simulink model "time_domain_exe2_not_autonomous"  (R2020b)
settings: Solver=VariableStepAuto  StartTime=0.0  StopTime=10.0  RelTol=1e-3
settings Model: Creator=petir  LastModifiedBy=petir

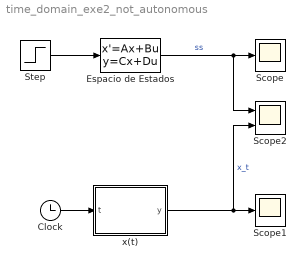
== system time_domain_exe2_not_autonomous ==
  Clock : Clock
  Espacio de Estados : StateSpace  A=[-5 0; 0 -5]  B=[5; 5]  C=[1, -1]  D=[0]  InitialCondition=[2; -1]
  Scope : Scope
  Scope1 : Scope
  Scope2 : Scope  NumInputPorts=2
  Step : Step  SampleTime=0
  x(t) : MATLAB Function  TreatAsAtomicUnit=on
  wires:
  Espacio de Estados/1 -> Scope2/1, Scope/1  "ss"
  Clock/1 -> x(t)/1(t)
  x(t)/1(y) -> Scope2/2, Scope1/1  "x_t"
  Step/1 -> Espacio de Estados/1

== matlab function time_domain_exe2_not_autonomous/x(t) ==
  data: t input; y output
function y = fcn(t)
x1 = 3*exp(-5*t);
y = x1;
